simulink model "AION_auto_unexpected_quit_analysis"  (R2021a)
settings: configuration reference "AION_IDS_Speedgoat" (kept outside this file)
settings Model: DataDictionary=AION_auto_unexpected_quit_analysis.sldd  Creator=Administrator  LastModifiedBy=Administrator
settings ConfigSetRef: SourceName=AION_IDS_Speedgoat

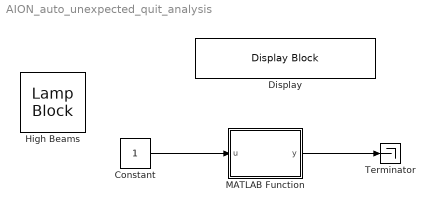
== system AION_auto_unexpected_quit_analysis ==
  Constant : Constant
  Display : DisplayBlock  LabelPosition=Hide  Transparency=1
  High Beams : LampBlock  Icon=HighBeams
  MATLAB Function : MATLAB Function  TreatAsAtomicUnit=on
  Terminator : Terminator
  wires:
  Constant/1 -> MATLAB Function/1(u)
  MATLAB Function/1(y) -> Terminator/1

== matlab function AION_auto_unexpected_quit_analysis/MATLAB Function ==
  data: u input; y output
function y = fcn(u)
% y = Active_status.ActiveStatus;
y = 1;
end
